simulink model "QEP_Test"  (R2025a)
settings: Solver=FixedStepAuto  StartTime=0.0  StopTime=20  RelTol=1e-3  EnableMultiTasking=on
undefined symbols (not defined in the file or in its folder): bit
libraries: c2802xlib x3
settings Model: ExtModeTrigDuration=8  Creator=mafur  LastModifiedBy=mafur
settings SolverCC: AutoInsertRateTranBlk=on
settings OptimizationCC: DefaultParameterBehavior=Inlined  DefaultUnderspecifiedDataType=single  EnhancedBackFolding=on  PassReuseOutputArgsAs=Individual arguments  MaxStackSize=1024  OptimizeBlockOrder=speed  DifferentSizesBufferReuse=on  OptimizationCustomize=off  EfficientTunableParamExpr=on
settings DebuggingCC: ParamPrecisionLossAbsoluteDiffThreshold=0.001  ParamPrecisionLossRelativeDiffThreshold=0.001  ParameterTunabilityLossMsg=error
settings HardwareCC: ProdBitPerChar=16.0  ProdBitPerInt=16.0  ProdBitPerPointer=32.0  ProdBitPerSizeT=32.0  ProdBitPerPtrDiffT=32.0  ProdLargestAtomicInteger=Integer  ProdLargestAtomicFloat=None  ProdWordSize=16.0  ProdLongLongMode=on  ProdHWDeviceType=Texas Instruments->C2000  HardwareBoardFeatureSet=SoCBlockset
settings RTWCC: SystemTargetFile=ert.tlc  HardwareBoard=TI Delfino F28379D LaunchPad  TemplateMakefile=ert_default_tmf  Toolchain=Texas Instruments Code Composer Studio (C2000)  CodeProfilingSaveOptions=MetricsOnly  Description=Embedded Coder
settings CodeAppCC: ForceParamTrailComments=on  IgnoreCustomStorageClasses=off  OperatorAnnotations=on  SimulinkDataObjDesc=on  SFDataObjDesc=on  InsertBlockDesc=on
settings ERTTargetCC: ExtModeTransport=4.0  ExtModeAutomaticAllocSize=off  ExtModeStaticAllocSize=10000.0  CodeReplacementLibrary=TI C28x

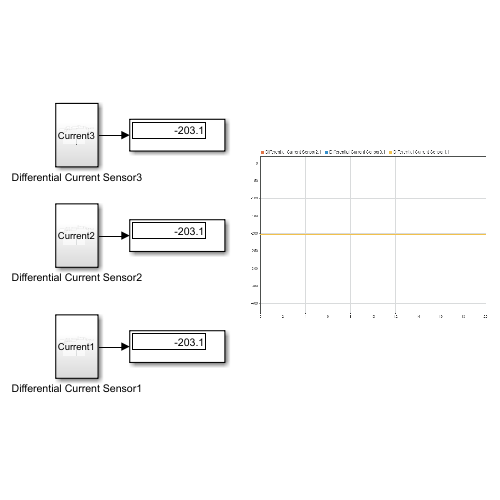
[thumbnail: Simulink's stored preview of the top-level diagram]
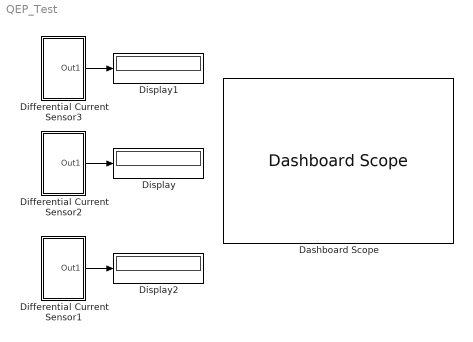
== system QEP_Test ==
  Dashboard Scope : DashboardScope  FontColor=[0.0, 0.0, 0.0]
  Differential Current Sensor1 : Subsystem
  Differential Current Sensor2 : Subsystem
  Differential Current Sensor3 : Subsystem
  Display : Display
  Display1 : Display
  Display2 : Display
  wires:
  Differential Current Sensor2/1(Out1) -> Display/1
  Differential Current Sensor3/1(Out1) -> Display1/1
  Differential Current Sensor1/1(Out1) -> Display2/1

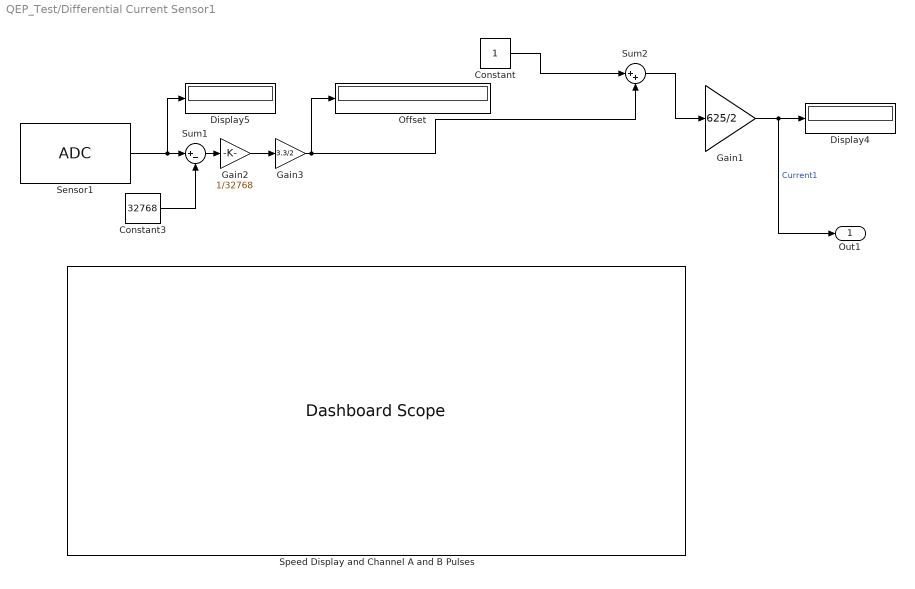
== system QEP_Test/Differential Current Sensor1 ==
  Constant : Constant
  Constant3 : Constant  Value=32768
  Display4 : Display
  Display5 : Display
  Gain1 : Gain  Gain=625/2
  Gain2 : Gain  Gain=1/32768
  Gain3 : Gain  Gain=3.3/2
  Offset : Display
  Sensor1 : c2802xlib/ADC  blkParamProc=C2000_Type4  ADCModule=D  samplingMode=Single sample mode  ADCResolution=16-bit (Differential inputs)  ADC29xResolution=12-bit  ADCMode=Single-ended input  useSOC1=SOC0  useSOC2=SOC0_SOC1  SOCAcquisitionWindow=15  SOCTriggerSource=Software  SOCInterruptTrigger=No ADCINT  Ts=0.001  dType=uint16  postInterrupt=off  interruptSel=ADCINT1  ADCINTContinuous=on  endma=off  chdma=1  conv1=ADCINA0  conv2=ADCINA0 and ADCINB0  conv1_Type4=ADCIN3  conv2_Type4=ADCIN14 and ADCIN15
      settings: LibrarySourceBlock=c2837xDlib/ADC
  Speed Display and Channel A and B Pulses : DashboardScope  FontColor=[0.0, 0.0, 0.0]
  Sum1 : Sum  Inputs=|+-
  Sum2 : Sum  Inputs=|++
  Out1 : Outport
  wires:
  Gain1/1 -> Out1/1, Display4/1  "Current1"
  Sensor1/1 -> Sum1/1, Display5/1
  Gain3/1 -> Sum2/2, Offset/1
  Sum1/1 -> Gain2/1
  Constant3/1 -> Sum1/2
  Gain2/1 -> Gain3/1
  Constant/1 -> Sum2/1
  Sum2/1 -> Gain1/1

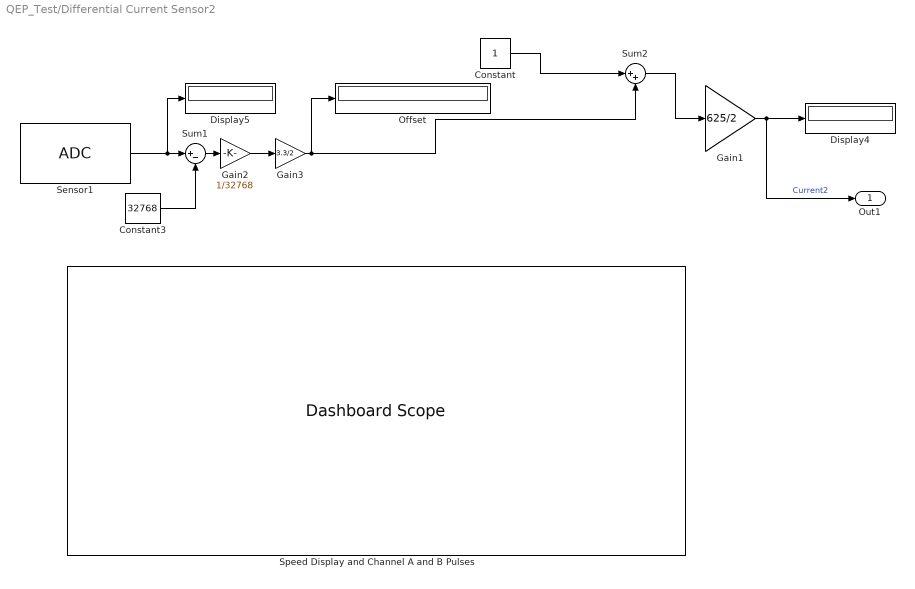
== system QEP_Test/Differential Current Sensor2 ==
  Constant : Constant
  Constant3 : Constant  Value=32768
  Display4 : Display
  Display5 : Display
  Gain1 : Gain  Gain=625/2
  Gain2 : Gain  Gain=1/32768
  Gain3 : Gain  Gain=3.3/2
  Offset : Display
  Sensor1 : c2802xlib/ADC  blkParamProc=C2000_Type4  ADCModule=D  samplingMode=Single sample mode  ADCResolution=16-bit (Differential inputs)  ADC29xResolution=12-bit  ADCMode=Single-ended input  useSOC1=SOC1  useSOC2=SOC0_SOC1  SOCAcquisitionWindow=15  SOCTriggerSource=Software  SOCInterruptTrigger=No ADCINT  Ts=0.001  dType=uint16  postInterrupt=off  interruptSel=ADCINT1  ADCINTContinuous=on  endma=off  chdma=1  conv1=ADCINA0  conv2=ADCINA0 and ADCINB0  conv1_Type4=ADCIN3  conv2_Type4=ADCIN12 and ADCIN13
      settings: LibrarySourceBlock=c2837xDlib/ADC
  Speed Display and Channel A and B Pulses : DashboardScope  FontColor=[0.0, 0.0, 0.0]
  Sum1 : Sum  Inputs=|+-
  Sum2 : Sum  Inputs=|++
  Out1 : Outport
  wires:
  Gain1/1 -> Out1/1, Display4/1  "Current2"
  Gain3/1 -> Sum2/2, Offset/1
  Constant3/1 -> Sum1/2
  Sum1/1 -> Gain2/1
  Constant/1 -> Sum2/1
  Gain2/1 -> Gain3/1
  Sum2/1 -> Gain1/1
  Sensor1/1 -> Sum1/1, Display5/1

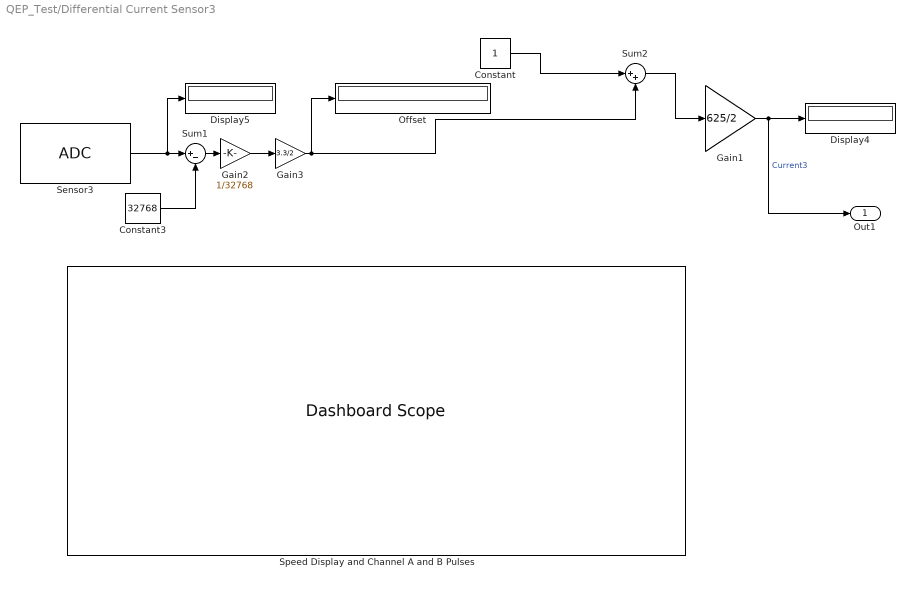
== system QEP_Test/Differential Current Sensor3 ==
  Constant : Constant
  Constant3 : Constant  Value=32768
  Display4 : Display
  Display5 : Display
  Gain1 : Gain  Gain=625/2
  Gain2 : Gain  Gain=1/32768
  Gain3 : Gain  Gain=3.3/2
  Offset : Display
  Sensor3 : c2802xlib/ADC  blkParamProc=C2000_Type4  ADCModule=D  samplingMode=Single sample mode  ADCResolution=16-bit (Differential inputs)  ADC29xResolution=12-bit  ADCMode=Single-ended input  useSOC1=SOC2  useSOC2=SOC0_SOC1  SOCAcquisitionWindow=15  SOCTriggerSource=Software  SOCInterruptTrigger=No ADCINT  Ts=0.001  dType=uint16  postInterrupt=off  interruptSel=ADCINT1  ADCINTContinuous=on  endma=off  chdma=1  conv1=ADCINA0  conv2=ADCINA0 and ADCINB0  conv1_Type4=ADCIN3  conv2_Type4=ADCIN10 and ADCIN11
      settings: LibrarySourceBlock=c2837xDlib/ADC
  Speed Display and Channel A and B Pulses : DashboardScope  FontColor=[0.0, 0.0, 0.0]
  Sum1 : Sum  Inputs=|+-
  Sum2 : Sum  Inputs=|++
  Out1 : Outport
  wires:
  Constant3/1 -> Sum1/2
  Gain3/1 -> Sum2/2, Offset/1
  Sum1/1 -> Gain2/1
  Sensor3/1 -> Sum1/1, Display5/1
  Sum2/1 -> Gain1/1
  Gain1/1 -> Out1/1, Display4/1  "Current3"
  Gain2/1 -> Gain3/1
  Constant/1 -> Sum2/1
